simulink model "AUAV_V3_TestSensors"  (R2015a)
settings: Solver=FixedStepDiscrete  StartTime=0.0  StopTime=10.0  FixedStep=T  RelTol=1e-3
PreLoadFcn:
  | %T = 0.0025;
  | MavlinkBus;
  | mcuInit;
  | % Baro Altitude Computation
  | % =========================
  | basePressure = 98192.64;
  | baseTemp = 288.215;
  | lapseRate = -0.00198122;
  | baseHeight = 0;
undefined symbols (not defined in the file): A0, A14, A15, A2, A3, A4, A5, A6, accBiasRateLimit, apSampleTime, B0, bankCommandLimit, barAdjust, baroCutoff, baroCutTemp, baroOffset, baroScale, barTGain1, barTGain2, barTMean1, barTMean2, bda, bde, bdr, bdt, bICda, bICde, bICdr, bICdt, cubeAccelGain16405, cubeGyroGain16405, cubeMagGain16405, D0, D11, D7, D8, daLimit, data, daTrimMax, daTrimMin, deLimit, derivativesConstant, deTrimMax, deTrimMin, drLimit, drTrimMax, drTrimMin, dtLimit, dtTrimMax, dtTrimMin, F2, F3, G0, G13, G15, gaind, GS_location, gyroBiasRateLimit, IC1max, imuOffset_xacc ... (+77)
libraries: MCHP_Blockset x158, simulink x84, SLUGS_Library x31, aerolibconvert2 x6, aerolibutil x4, aerolibtransform2 x3, dspmtrx3 x2, aerolibobsolete x2
(part 13 of 23)

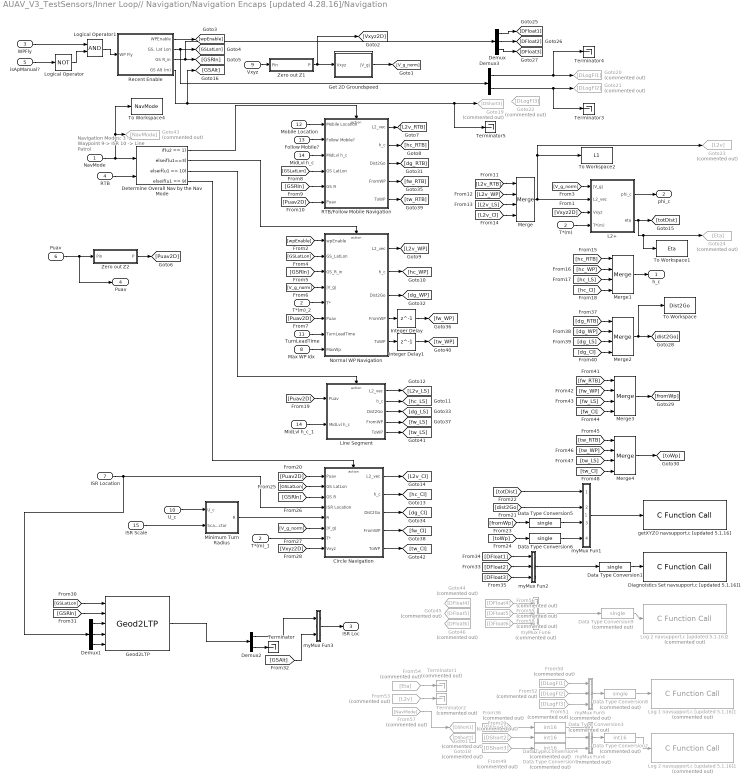
== system AUAV_V3_TestSensors/Inner Loop// Navigation/Navigation Encaps [updated 4.28.16]/Navigation ==
  note: Navigation Modes:
      | 3 -> Waypoint
      | 9-> ISR
      | 10 -> Line Patrol
  NavMode : Inport
  T*(m) : Inport  Port=2
  WPFly : Inport  Port=3
  RTB : Inport  Port=4
  isApManual? : Inport  Port=5
  Puav : Inport  Port=6  SampleTime=apSampleTime
  ISR Location : Inport  Port=7
  Max WP Idx : Inport  Port=8
  Vxyz : Inport  Port=9  SampleTime=apSampleTime
  U_c : Inport  Port=10
  TurnLeadTime : Inport  Port=11
  Mobile Location : Inport  Port=12
  Follow Mobile? : Inport  Port=13
  MidLvl h_c : Inport  Port=14
  ISR Scale : Inport  Port=15
  Circle Navigation : Subsystem  TreatAsAtomicUnit=on
  Data Type Conversion1 : DataTypeConversion  OutDataTypeStr=single
  Data Type Conversion{2..4,7} (4 alike) : DataTypeConversion  Commented=on  OutDataTypeStr=int16
  Data Type Conversion5 : DataTypeConversion  OutDataTypeStr=single
  Data Type Conversion6 : DataTypeConversion  OutDataTypeStr=single
  Data Type Conversion8 : DataTypeConversion  Commented=on  OutDataTypeStr=single
  Data Type Conversion9 : DataTypeConversion  Commented=on  OutDataTypeStr=single
  Demux : Demux  Outputs=3
  Demux1 : Demux  Outputs=3
  Demux2 : Demux  Outputs=[2 1]
  Demux3 : Demux  Outputs=2
  Determine Overall Nav by the Nav Mode : If  NumInputs=2  IfExpression=u2 == 1  ElseIfExpressions=u1==3, u1 == 10, u1 == 9  ShowElse=off
  Diagnoistics Set navsupport.c [updated 5.1.16]1 : MCHP_Blockset/User Functions/C Function Call  ParseFilesChkbx=off  ListFunctions1=Custom Function  Function1=void setDiagnosticFloat(float * flValues)  AddHeaderDeclaration=on  Function1Type=when block is updated (default)  Fct1BlockIn=flValues  FctReturnBlockOut=on  DataCollected=0  ORDERING=None  SampleTime=-1  MCHP_MASTERLINK=|  PinDigitalInput=[]  PinDigitalOutput=[]  PinAnalogInput=[]
      | AUAV_V3_TestSensors/Microchip Master
      | AUAV V3 Board
      | Busy Flag on D2 (RA6)
  From29 : From  Commented=on  GotoTag=DShort2
  From36 : From  Commented=on  GotoTag=DShort1
  From49 : From  Commented=on  GotoTag=DShort3
  From50 : From  Commented=on  GotoTag=DLogFl1
  From51 : From  Commented=on  GotoTag=DLogFl3
  From52 : From  Commented=on  GotoTag=DLogFl2
  From53 : From  Commented=on  GotoTag=L2v
  From54 : From  Commented=on  GotoTag=Eta
  From55 : From  Commented=on  GotoTag=DFloat5
  From56 : From  Commented=on  GotoTag=DFloat4
  From57 : From  Commented=on  GotoTag=NavMode
  From58 : From  Commented=on  GotoTag=DFloat6
  Geod2LTP : SLUGS_Library/Navigation/Geod2LTP
  Get 2D Groundspeed : Subsystem
  Goto17 : Goto  Commented=on  GotoTag=DShort1
  Goto18 : Goto  Commented=on  GotoTag=DShort2
  Goto19 : Goto  Commented=on  GotoTag=DShort3
  Goto20 : Goto  Commented=on  GotoTag=DLogFl1
  Goto21 : Goto  Commented=on  GotoTag=DLogFl2
  Goto22 : Goto  Commented=on  GotoTag=DLogFl3
  Goto23 : Goto  Commented=on  GotoTag=L2v
  Goto24 : Goto  Commented=on  GotoTag=Eta
  Goto43 : Goto  Commented=on  GotoTag=NavMode
  Goto44 : Goto  Commented=on  GotoTag=DFloat4
  Goto45 : Goto  Commented=on  GotoTag=DFloat5
  Goto46 : Goto  Commented=on  GotoTag=DFloat6
  Integer Delay : Delay  DelayLength=1  InputProcessing=Inherited
  Integer Delay1 : Delay  DelayLength=1  InputProcessing=Inherited
  L2+ : Subsystem
  Line Segment : Subsystem  TreatAsAtomicUnit=on
  Log 1 navsupport.c [updated 5.1.16]1 : MCHP_Blockset/User Functions/C Function Call  Commented=on  ParseFilesChkbx=off  ListFunctions1=Custom Function  Function1=void setDiagnosticFloat(float * flValues)  AddHeaderDeclaration=on  Function1Type=when block is updated (default)  Fct1BlockIn=flValues  FctReturnBlockOut=on  DataCollected=0  ORDERING=None  SampleTime=-1  MCHP_MASTERLINK=|  PinDigitalInput=[]  PinDigitalOutput=[]  PinAnalogInput=[]
      | AUAV_V3_TestSensors/Microchip Master
      | AUAV V3 Board
      | Busy Flag on D2 (RA6)
  Log 2 navsupport.c [updated 5.1.16]1 : MCHP_Blockset/User Functions/C Function Call  Commented=on  ParseFilesChkbx=off  ListFunctions1=Custom Function  Function1=void setDiagnosticShort(int16_t *shValues)  AddHeaderDeclaration=on  Function1Type=when block is updated (default)  Fct1BlockIn=shValues  FctReturnBlockOut=on  DataCollected=0  ORDERING=None  SampleTime=-1  MCHP_MASTERLINK=|  PinDigitalInput=[]  PinDigitalOutput=[]  PinAnalogInput=[]
      | AUAV_V3_TestSensors/Microchip Master
      | AUAV V3 Board
      | Busy Flag on D2 (RA6)
  Log 2 navsupport.c [updated 5.1.16]2 : MCHP_Blockset/User Functions/C Function Call  Commented=on  ParseFilesChkbx=off  ListFunctions1=Custom Function  Function1=void setDiagnosticFloat(float * flValues)  AddHeaderDeclaration=on  Function1Type=when block is updated (default)  Fct1BlockIn=flValues  FctReturnBlockOut=on  DataCollected=0  ORDERING=None  SampleTime=-1  MCHP_MASTERLINK=|  PinDigitalInput=[]  PinDigitalOutput=[]  PinAnalogInput=[]
      | AUAV_V3_TestSensors/Microchip Master
      | AUAV V3 Board
      | Busy Flag on D2 (RA6)
  Logical Operator : Logic  Operator=NOT  AllPortsSameDT=off  OutDataTypeStr=boolean
  Logical Operator1 : Logic  AllPortsSameDT=off  OutDataTypeStr=boolean
  Merge{,1..4} (5 alike) : Merge  Inputs=4
  MidLvl h_c_1 : InportShadow  Port=14
  Minimum Turn Radius : Subsystem
  Normal WP Navigation : Subsystem  TreatAsAtomicUnit=on
  RTB/Follow Mobile Navigation : Subsystem
  Recent Enable : Subsystem
  T*(m)_1 : InportShadow  Port=2
  T*(m)_2 : InportShadow  Port=2
  Terminator{,3..5} (4 alike) : Terminator
  Terminator1 : Terminator  Commented=on
  Terminator2 : Terminator  Commented=on
  To Workspace : ToWorkspace  VariableName=Dist2Go  SampleTime=-1
  To Workspace1 : ToWorkspace  VariableName=Eta  SampleTime=-1
  To Workspace2 : ToWorkspace  VariableName=L1  SampleTime=-1
  To Workspace4 : ToWorkspace  VariableName=NavMode  SampleTime=-1
  Zero out Z1 : MATLAB Function  TreatAsAtomicUnit=on
  Zero out Z2 : MATLAB Function  TreatAsAtomicUnit=on
  getXYZ() navsupport.c [updated 5.1.16] : MCHP_Blockset/User Functions/C Function Call  ParseFilesChkbx=on  ListFunctions1=Custom Function  Function1=void setNavNav(float* values)  AddHeaderDeclaration=on  Function1Type=when block is updated (default)  Fct1BlockIn=values  FctReturnBlockOut=on  DataCollected="s.chksm=reshape({ '638529-אוק-2016 01:00:36','251929-אוק-2016 01:00:36','1689429-אוק-2016 01:00:36','4250714-אוק-2016 08:45:05','360329-אוק-2016 01:00:36','7293729-אוק-2016 01:00:36','954929-אוק-2016 01:00:36','296129-אוק-2016 01:00:36','278129-אוק-2016 01:00:36','556029-אוק-2016 01:00:36','963229-אוק-2016 01:00:36','1122729-אוק-2016 01:00:36','372429-אוק-2016 01:00:36','998829-אוק-2016 01:00:36','536514-אוק-2016 08:45:05'},1,15);s.File1=reshape({ '  void  newCircBuffer(CBRef cB)','  void  freeCircBuffer(CBRef* cB)','  void  freeCircBuffer(CBRef* cB)',' unsigned int  getLength(CBRef cB)','  int  readHead(CBRef cB)','  int  readTail(CBRef cB)',' unsigned char  peak(CBRef cB)',' unsigned char  readFront(CBRef cB)',' unsigned char  writeBack(CBRef cB, unsigned char data)','  void  makeEmpty(CBRef cB)','  void  printCircBuf(CBRef cB)'},1,11);s.File2=reshape({ '  void  uartBufferInit(void)','  void  __attribute__((__interrupt__, no_auto_psv)) _U4RXInterrupt(void)','  void  getGPSRawData(unsigned char* gpsBuffer)',' unsigned char  isGPSNovatel(void)'},1,4);s.File3=reshape({ '  char  hex2char(char halfhex)','  float  degMinToDeg(unsigned char degrees, float minutes)',' unsigned char  gpsUbloxSeparate(unsigned char* outStream)','  void  gpsUbloxParse(void)','  void  getGpsUbloxMainData(float* data)','  void  getGpsUbloxData(float* data)','  char  gpSmbl(char symbl)',' unsigned char  myTokenizer(char* stringToTokenize, char token, char * returnToken)','  void  parseRMC(unsigned char* stream)','  void  parseGGA(unsigned char* stream)',' unsigned char  getChecksum(unsigned char* sentence, unsigned char size)','  void  gpsDebugMsg(unsigned char buf)'},1,12);s.File4=reshape({ '  void  uartMavlinkBufferInit(void)','  void __attribute__((__interrupt__,__auto_psv__)) _U1RXInterrupt(void)','  uint8_t  isFinite(float s)','  void  InitParameterInterface(void)','  void  protDecodeMavlink(void)','  uint16_t  MissionInterfaceResponse(uint8_t system_id, uint8_t component_id)','  uint16_t  ParameterInterfaceResponse(uint8_t system_id, uint8_t component_id)','  uint16_t  PackHeartBeat(uint8_t system_id, uint8_t component_id)','  uint16_t  PackTextMsg(uint8_t system_id, uint8_t component_id, unsigned char buf)','  uint16_t  PackRawIMU(uint8_t system_id, uint8_t component_id, mavlink_raw_imu_t mlRawIMUData ,uint32_t time_usec)','  uint16_t  PackRawAttitude(uint8_t system_id, uint8_t component_id, mavlink_attitude_t mlAttitudeData ,uint32_t time_usec)','  uint16_t  PackPosXYZ_Sol(uint8_t system_id, uint8_t component_id, mavlink_local_position_ned_t mlLocalPositionSol ,uint32_t time_usec)','  uint16_t  PackGpsRawInt(uint8_t system_id, uint8_t component_id, mavlink_gps_raw_int_t mlRawGpsDataInt ,uint32_t time_usec)','  uint16_t  PackScaledPressure(uint8_t system_id, uint8_t component_id, mavlink_scaled_pressure_t mlAirData ,uint32_t time_usec)','  uint16_t  PackSysStatus(uint8_t system_id, uint8_t component_id, mavlink_sys_status_t mlSysStatus)','  uint16_t  PackRawServo(uint8_t system_id, uint8_t component_id, mavlink_servo_output_raw_t mlPwmCommands ,uint32_t time_usec)','  uint16_t  HIL_PackRawServo(uint8_t system_id, uint8_t component_id, mavlink_servo_output_raw_t mlPwmCommands ,uint32_t time_usec)','  uint16_t  PackRawRC(uint8_t system_id, uint8_t component_id, mavlink_rc_channels_raw_t mlRC_Commands ,uint32_t time_usec)','  uint16_t  PackVFR_HUD(uint8_t system_id, uint8_t component_id, mavlink_vfr_hud_t mlVfr_hud ,uint32_t time_usec)','  char  sendQGCDebugMessage(const char * dbgMessage, char severity, unsigned char* bytesToAdd, char positionStart)','  void  TxN_Data_OverU1(uint16_t N)','  void  TxN_Data_OverU4(uint16_t N)'},1,22);s.File5=reshape({ '  float  myAtan2(float num, float denom)','  float  myPow(float x, float toTheN)','  float  mySqrt(float x)','  float  myAbs(float x)','  float  myAtan(float x)','  float  myAsin(float x)','  float  mySin(float x)','  float  myCos(float x)','  float  myTan(float x)','  float  myAcos(float x)','  float  myExp(float x)','  void  hugeDelay(void)','  void  smallDelay(void)','  void  tinyDelay(void)','  void  printToUart2(const char *fmt, ...)'},1,15);s.File6=reshape({ '  void  sendTelemetryMavlink(unsigned char* dataOut)','  void  uart2Init(void)','  void  gsRead(unsigned char* gsChunk)','  void  prepareTelemetryMavlink(unsigned char* dataOut)','  void  prepareTelemetryMavlink(unsigned char* dataOut)','  void  sendTelemetryMavlink(unsigned char* dataOut)','  void  copyBufferToDMA1(unsigned char size)','  void  send2GS(unsigned char* protData)','  uint8_t  clearWaypointsFrom(uint8_t startingWp)','  void  addMessageToSpiOut(mavlink_message_t* msg)'},1,10);s.File7={ '  void  populateParameterInterface(void)'};s.File8={ '  void  mavlinkInit(void)'};s.File9=reshape({ '  void  updatePWM(unsigned short * PWMData)','  void  updatePWMTrim(unsigned short PWMData, unsigned char channel)','  void  updateLoad(uint8_t mcuLoad)','  void  updateEuler(float* newEuler)','  void  updatePQR(float* newPQR)',' unsigned char  getHilOnOff(void)','  uint8_t  getLightsOnOff(void)','  uint8_t  getLightsDayNight(void)','  void  updateVISensor(uint16_t* data)','  void  updatePTZ(int16_t* ptz)'},1,10);s.File10=reshape({ '  void  updateRawADCData(int16_t* adcData)','  void  updateAirData(float* airData)','  void  updateLoadData(uint8_t load, uint16_t mvPower)','  void  updateAttitude(float * attitudeData)','  void  getGSLocation(float* altLatLon)','  void  updateTimeStamp(uint32_t timeSt)','  void  updatePosition(float * posData)','  void  updatePilotConsole(uint16_t * pilData)','  void  updateDiagnosticFl(float* diagFl)','  void  updateDiagnosticSh(int16_t* diagSh)','  void  updateBias(float * biasData)','  void  updateSensorData(float* sens)','  uint8_t  isFixValid(void)','  void  updateSensorDiag(float* diag)'},1,14);s.File11=reshape({ '  void  gpsInit(void)','  void  gpsParse(uint8_t* dataStream)','  void  updateStatus(uint8_t* completeMessage)','  void  updatePositionData(uint8_t* completeMessage)','  void  updateVelocityData(uint8_t* completeMessage)','  void  updateTimeData(uint8_t* completeMessage)','  void  getGpsMainData(float* data)','  uint32_t  CRC32Value(int32_t i)','  uint32_t  CalculateBlockCRC32(uint32_t ulCount, uint8_t *ucBuffer)','  uint16_t  charsToUint16(uint8_t* data)','  uint32_t  charsToUint32(uint8_t* data)','  float  charsToFloat(uint8_t* data)','  double  charsToDouble(uint8_t* data)'},1,13);s.File12=reshape({ '  void  getMidLevelCommands(float* commands)',' unsigned char  isApManual(uint16_t failsafe)','  float  getParamIdx(unsigned char idx)','  void  getRangeOfParams(uint8_t startIdx, uint8_t endIdx, float* parameters)','  float  getDynamic(void)','  void  getAttitude(float* attitude)','  void  getXYZ(float* xyz)','  void  getVned(float* xyz)','  uint8_t  getMaxWp(void)',' unsigned char  isWpFly(void)',' unsigned char  isPassthrough(void)','  void  setDiagnosticFloat(float * flValues)','  void  setDiagnosticShort(int16_t* shValues)','  void  getWP(unsigned char idx, float* WPpos)','  void  setLogFloat1(float * flValues)','  void  setLogFloat2(float * flValues)',' unsigned char  getApControlType(void)',' unsigned char  getPassValues(uint8_t* pasVals)','  void  setCurrentCommands(float airSpeed)','  void  getCurrentGPSPos(float* latLonAlt)','  void  setNavLong(float* values)','  void  setNavLat(float* values)','  void  setNavNav(float* values)','  void  getAccels(float * accels)','  void  getAccBias(float * bias)','  void  getRTB(uint8_t* rtb)','  void  getMobileLocation(float* loc)','  uint8_t  getNavMode(void)','  void  getISRLocation(float* loc)','  uint8_t  getISRCameraOption1(void)',' unsigned short  meanFilter5(unsigned short * values)','  uint8_t  justEnabled(uint8_t enableValue, uint8_t index)',' unsigned char  quickSort(unsigned short *arr, char elements)'},1,33);s.File13=reshape({ '  void  hilRead(unsigned char* hilChunk)','  void  hil_getRawRead(short * rawData)','  void  hil_getVned(float* vned)','  void  hil_getEuler(float* euler)','  void  hil_getRates(float* pqr)','  void  hil_getXYZ(float* xyz)',' unsigned int  hil_getTs(void)','  void  protDecodeHil(uint8_t* dataIn)'},1,8);s.File14=reshape({ '  void  cubeInit(void)','  void  getCubeData(short * cubeData)','  void  updateCubeData(void)','  int16_t  averageData(int16_t* theData, uint8_t count)',' unsigned short  write2Cube(unsigned short data2Send)','  short  convert14BitToShort(short wordData)','  short  convert12BitToShort(short wordData)',' unsigned char  isCube16405(void)'},1,8);s.File15=reshape({ '  void  uartMavlinkBufferInit(void)','  uint16_t  PackHeartBeat(uint8_t system_id, uint8_t component_id)','  uint16_t  PackRawServo(uint8_t system_id, uint8_t component_id, mavlink_servo_output_raw_t mlPwmCommands ,uint32_t time_usec)','  uint16_t  HIL_PackRawServo(uint8_t system_id, uint8_t component_id, mavlink_servo_output_raw_t mlPwmCommands ,uint32_t time_usec)','  uint16_t  PackRawRC(uint8_t system_id, uint8_t component_id, mavlink_rc_channels_raw_t mlRC_Commands, uint32_t time_usec)','  uint16_t  PackVFR_HUD(uint8_t system_id, uint8_t component_id, mavlink_vfr_hud_t mlVfr_hud, uint32_t time_usec)','  uint16_t  PackRawIMU(uint8_t system_id, uint8_t component_id, mavlink_raw_imu_t mlRawIMUData ,uint32_t time_usec)','  uint16_t  PackRawAttitude(uint8_t system_id, uint8_t component_id, mavlink_attitude_t mlAttitudeData ,uint32_t time_usec)','  uint16_t  PackPosXYZ_Sol(uint8_t system_id, uint8_t component_id, mavlink_local_position_ned_t mlLocalPositionSol ,uint32_t time_usec)','  char  sendQGCDebugMessage(const char * dbgMessage, char severity, unsigned char* bytesToAdd, char positionStart)','  uint16_t  PackGpsRawInt(uint8_t system_id, uint8_t component_id, mavlink_gps_raw_int_t mlRawGpsDataInt, uint32_t time_usec)','  uint16_t  PackScaledPressure(uint8_t system_id, uint8_t component_id, mavlink_scaled_pressure_t mlAirData, uint32_t time_usec)','  uint16_t  PackSysStatus(uint8_t system_id, uint8_t component_id, mavlink_sys_status_t mlSysStatus)'},1,13);"  ORDERING=None  SampleTime=-1  MCHP_MASTERLINK=|  PinDigitalInput=[]  PinDigitalOutput=[]  PinAnalogInput=[]
      | AUAV_V3_TestSensors/Microchip Master
      | AUAV V3 Board
      | Busy Flag on D2 (RA6)
  myMux Fun1 : MATLAB Function  TreatAsAtomicUnit=on
  myMux Fun2 : MATLAB Function  TreatAsAtomicUnit=on
  myMux Fun3 : MATLAB Function  TreatAsAtomicUnit=on
  myMux Fun4 : MATLAB Function  Commented=on  TreatAsAtomicUnit=on
  myMux Fun5 : MATLAB Function  Commented=on  TreatAsAtomicUnit=on
  myMux Fun6 : MATLAB Function  Commented=on  TreatAsAtomicUnit=on
  h_c : Outport
  phi_c : Outport  Port=2
  ISR Loc : Outport  Port=3
  "Puav " : Outport  Port=4
  wires:
  Data Type Conversion8/1 -> Log 1 navsupport.c [updated 5.1.16]1/1
  From50/1 -> myMux Fun5/1(u1)
  From52/1 -> myMux Fun5/2(u2)
  From51/1 -> myMux Fun5/3(u3)
  myMux Fun5/1(y) -> Data Type Conversion8/1
  Data Type Conversion7/1 -> myMux Fun4/3(u3)
  Data Type Conversion4/1 -> myMux Fun4/2(u2)
  Data Type Conversion3/1 -> myMux Fun4/1(u1)
  From49/1 -> Data Type Conversion7/1
  From36/1 -> Data Type Conversion3/1
  From29/1 -> Data Type Conversion4/1
  myMux Fun4/1(y) -> Data Type Conversion2/1
  Data Type Conversion2/1 -> Log 2 navsupport.c [updated 5.1.16]1/1
  [GSAlt] -> myMux Fun3/2(u2)
  Geod2LTP/1 -> Demux2/1
  Demux2/2 -> Terminator/1
  Demux2/1 -> myMux Fun3/1(u1)
  myMux Fun3/1(y) -> ISR Loc/1
  [GSRIn] -> Geod2LTP/2
  [GSLatLon] -> Geod2LTP/1
  Demux1/3 -> Geod2LTP/5
  Demux1/2 -> Geod2LTP/4
  Demux1/1 -> Geod2LTP/3
  Data Type Conversion1/1 -> Diagnoistics Set navsupport.c [updated 5.1.16]1/1
  [DFloat3] -> myMux Fun2/3(u3)
  [DFloat1] -> myMux Fun2/1(u1)
  [DFloat2] -> myMux Fun2/2(u2)
  ISR Scale/1 -> Minimum Turn Radius/2(Scale Factor)
  U_c/1 -> Minimum Turn Radius/1(U_c)
  ISR Location/1 -> Demux1/1, Circle Navigation/4(ISR Location)
  [Vxyz2D] -> Circle Navigation/8(Vxyz)
  T*(m)_1/1 -> Circle Navigation/7(T*)
  [V_g_norm] -> Circle Navigation/6(|V_g|)
  Minimum Turn Radius/1(R) -> Circle Navigation/5(R)
  [GSRIn] -> Circle Navigation/3(GS R)
  [GSLatLon] -> Circle Navigation/2(GS LatLon)
  Circle Navigation/5(ToWP) -> [tw_CI]
  Circle Navigation/4(FromWP) -> [fw_CI]
  Circle Navigation/3(Dist2Go) -> [dg_CI]
  Circle Navigation/1(L2_vec) -> [L2v_CI]
  Circle Navigation/2(h_c) -> [hc_CI]
  [Puav2D] -> Circle Navigation/1(Puav)
  Integer Delay1/1 -> [tw_WP]
  Integer Delay/1 -> [fw_WP]
  Line Segment/5(ToWP) -> [tw_LS]
  Normal WP Navigation/5(ToWP) -> Integer Delay1/1
  RTB/Follow Mobile Navigation/5(ToWP) -> [tw_RTB]
  Line Segment/4(FromWP) -> [fw_LS]
  Normal WP Navigation/4(FromWP) -> Integer Delay/1
  RTB/Follow Mobile Navigation/4(FromWP) -> [fw_RTB]
  Line Segment/3(Dist2Go) -> [dg_LS]
  Normal WP Navigation/3(Dist2Go) -> [dg_WP]
  RTB/Follow Mobile Navigation/3(Dist2Go) -> [dg_RTB]
  Merge3/1 -> [fromWp]
  Merge4/1 -> [toWp]
  Merge2/1 -> [dist2Go], To Workspace/1
  [tw_RTB] -> Merge4/1
  [tw_WP] -> Merge4/2
  [tw_LS] -> Merge4/3
  [tw_CI] -> Merge4/4
  [fw_RTB] -> Merge3/1
  [fw_WP] -> Merge3/2
  [fw_LS] -> Merge3/3
  [fw_CI] -> Merge3/4
  [dg_RTB] -> Merge2/1
  [dg_WP] -> Merge2/2
  [dg_LS] -> Merge2/3
  [dg_CI] -> Merge2/4
  L2+/2(eta) -> [totDist], Goto24/1, To Workspace1/1
  Data Type Conversion6/1 -> myMux Fun1/4(u4)
  Data Type Conversion5/1 -> myMux Fun1/3(u3)
  [toWp] -> Data Type Conversion6/1
  [fromWp] -> Data Type Conversion5/1
  [dist2Go] -> myMux Fun1/2(u2)
  [totDist] -> myMux Fun1/1(u1)
  myMux Fun1/1(y) -> getXYZ() navsupport.c [updated 5.1.16]/1
  Vxyz/1 -> Zero out Z1/1(Pin)
  Get 2D Groundspeed/1(|V_g|) -> [V_g_norm]
  [Vxyz2D] -> L2+/3(Vxyz)
  [V_g_norm] -> L2+/1(|V_g|)
  L2+/1(phi_c) -> phi_c/1
  T*(m)/1 -> L2+/4(T*(m))
  NavMode/1 -> Determine Overall Nav by the Nav Mode/1, Goto43/1, To Workspace4/1
  Merge/1 -> L2+/2(L2_vec), Goto23/1, To Workspace2/1
  Recent Enable/1(WPEnable) -> [wpEnable]
  Recent Enable/2("GS, Lat Lon") -> [GSLatLon], Demux3/1
  Recent Enable/3(GS R_in) -> [GSRIn], Demux/1
  RTB/1 -> Determine Overall Nav by the Nav Mode/2
  Follow Mobile?/1 -> RTB/Follow Mobile Navigation/2(Follow Mobile?)
  MidLvl h_c/1 -> RTB/Follow Mobile Navigation/3(MidLvl h_c)
  Mobile Location/1 -> RTB/Follow Mobile Navigation/1(Mobile Location)
  Zero out Z1/1(P) -> Get 2D Groundspeed/1(Vxyz), [Vxyz2D]
  Puav/1 -> "Puav "/1, Zero out Z2/1(Pin)
  [GSRIn] -> Normal WP Navigation/3(GS_R_in)
  [GSLatLon] -> Normal WP Navigation/2(GS_LatLon)
  [wpEnable] -> Normal WP Navigation/1(wpEnable)
  [V_g_norm] -> Normal WP Navigation/4(|V_g|)
  T*(m)_2/1 -> Normal WP Navigation/5(T*)
  [Puav2D] -> Normal WP Navigation/6(Puav)
  TurnLeadTime/1 -> Normal WP Navigation/7(TurnLeadTime)
  Max WP Idx/1 -> Normal WP Navigation/8(MaxWp)
  [GSLatLon] -> RTB/Follow Mobile Navigation/4(GS LatLon)
  [GSRIn] -> RTB/Follow Mobile Navigation/5(GS R)
  Zero out Z2/1(P) -> [Puav2D]
  [Puav2D] -> RTB/Follow Mobile Navigation/6(Puav)
  Merge1/1 -> h_c/1
  RTB/Follow Mobile Navigation/1(L2_vec) -> [L2v_RTB]
  RTB/Follow Mobile Navigation/2(h_c) -> [hc_RTB]
  Normal WP Navigation/1(L2_vec) -> [L2v_WP]
  Normal WP Navigation/2(h_c) -> [hc_WP]
  Line Segment/1(L2_vec) -> [L2v_LS]
  Line Segment/2(h_c) -> [hc_LS]
  [L2v_RTB] -> Merge/1
  [L2v_WP] -> Merge/2
  [L2v_LS] -> Merge/3
  [L2v_CI] -> Merge/4
  [hc_RTB] -> Merge1/1
  [hc_WP] -> Merge1/2
  [hc_LS] -> Merge1/3
  [hc_CI] -> Merge1/4
  [Puav2D] -> Line Segment/1(Puav)
  MidLvl h_c_1/1 -> Line Segment/2(MidLvl h_c)
  isApManual?/1 -> Logical Operator/1
  Logical Operator1/1 -> Recent Enable/1(WP Fly)
  Logical Operator/1 -> Logical Operator1/2
  WPFly/1 -> Logical Operator1/1
  myMux Fun2/1(y) -> Data Type Conversion1/1
  From54/1 -> Terminator1/1
  From53/1 -> Terminator2/1
  Demux/1 -> [DFloat1]
  Demux/2 -> [DFloat2]
  Demux3/1 -> Terminator4/1, Goto20/1
  Demux3/2 -> Terminator3/1, Goto21/1
  From57/1 -> Goto17/1
  Demux/3 -> [DFloat3]
  Recent Enable/4(GS Alt (m)) -> Terminator5/1, Goto19/1, [GSAlt]
  From58/1 -> myMux Fun6/3(u3)
  From56/1 -> myMux Fun6/1(u1)
  From55/1 -> myMux Fun6/2(u2)
  myMux Fun6/1(y) -> Data Type Conversion9/1
  Data Type Conversion9/1 -> Log 2 navsupport.c [updated 5.1.16]2/1
  Determine Overall Nav by the Nav Mode/1 -> RTB/Follow Mobile Navigation/Action
  Determine Overall Nav by the Nav Mode/2 -> Normal WP Navigation/Action
  Determine Overall Nav by the Nav Mode/3 -> Line Segment/Action
  Determine Overall Nav by the Nav Mode/4 -> Circle Navigation/Action

== system AUAV_V3_TestSensors/Position_and_Attitude_Filter/Attitude Complimentary Filter COG/3D Filter ==
  In1 : Inport
  Data Type Conversion1 : DataTypeConversion  OutDataTypeStr=single
  Data Type Conversion2 : DataTypeConversion  OutDataTypeStr=double
  Demux : Demux  Outputs=3
  Filter1 : Subsystem  mask(DiscretizedZeroPole){Zeros=zval, Poles=pval, Gain=kval, AbsTol=auto, SampleTime=TSample, method=tustin, Wc=1}
      mask prompts: Zeros "Zeros (enter in s-main:)"; Poles "Poles (enter in s-domain:)"; Gain "Gain (enter in s-domain:)"; AbsTol "Absolute tolerance:"; SampleTime "Sample time:"; Wc "Critical Frequency (Hz):"
      mask help: Continuous mask uses c2d to transform parameters onto the Discrete Zero-Pole block inside.
      mask init: same as AUAV_V3_TestSensors/Barometer_Driver/Baro Altimeter/Initial Baro Bias/Low Pass8
      mask TypeOptions method: zoh | foh | tustin | prewarp | matched
      mask Callback method: hidecrit
      mask Display:
      | droots(zeross,poless,gainss)
      | text( 0.5, 1.0, method, 'verticalAlignment','top')
  Filter2 : Subsystem  mask(DiscretizedZeroPole){Zeros=zval, Poles=pval, Gain=kval, AbsTol=auto, SampleTime=TSample, method=tustin, Wc=1}
      mask prompts: Zeros "Zeros (enter in s-main:)"; Poles "Poles (enter in s-domain:)"; Gain "Gain (enter in s-domain:)"; AbsTol "Absolute tolerance:"; SampleTime "Sample time:"; Wc "Critical Frequency (Hz):"
      mask help: Continuous mask uses c2d to transform parameters onto the Discrete Zero-Pole block inside.
      mask init: same as AUAV_V3_TestSensors/Barometer_Driver/Baro Altimeter/Initial Baro Bias/Low Pass8
      mask TypeOptions method: zoh | foh | tustin | prewarp | matched
      mask Callback method: hidecrit
      mask Display:
      | droots(zeross,poless,gainss)
      | text( 0.5, 1.0, method, 'verticalAlignment','top')
  Filter3 : Subsystem  mask(DiscretizedZeroPole){Zeros=zval, Poles=pval, Gain=kval, AbsTol=auto, SampleTime=TSample, method=tustin, Wc=1}
      mask prompts: Zeros "Zeros (enter in s-main:)"; Poles "Poles (enter in s-domain:)"; Gain "Gain (enter in s-domain:)"; AbsTol "Absolute tolerance:"; SampleTime "Sample time:"; Wc "Critical Frequency (Hz):"
      mask help: Continuous mask uses c2d to transform parameters onto the Discrete Zero-Pole block inside.
      mask init: same as AUAV_V3_TestSensors/Barometer_Driver/Baro Altimeter/Initial Baro Bias/Low Pass8
      mask TypeOptions method: zoh | foh | tustin | prewarp | matched
      mask Callback method: hidecrit
      mask Display:
      | droots(zeross,poless,gainss)
      | text( 0.5, 1.0, method, 'verticalAlignment','top')
  myMux Fun1 : MATLAB Function  TreatAsAtomicUnit=on
  Out1 : Outport
  wires:
  myMux Fun1/1(y) -> Data Type Conversion1/1
  In1/1 -> Data Type Conversion2/1
  Filter3/1(Out1) -> myMux Fun1/3(u3)
  Filter2/1(Out1) -> myMux Fun1/2(u2)
  Filter1/1(Out1) -> myMux Fun1/1(u1)
  Demux/3 -> Filter3/1(In1)
  Demux/2 -> Filter2/1(In1)
  Demux/1 -> Filter1/1(In1)
  Data Type Conversion2/1 -> Demux/1
  Data Type Conversion1/1 -> Out1/1

== system AUAV_V3_TestSensors/Position_and_Attitude_Filter/Attitude Complimentary Filter COG/Deriv  ==
  y : Inport
  Gain2 : Gain  Gain=[ 1/(5*apSampleTime) ]
  Integer Delay1 : Delay  DelayLength=5  InitialCondition=double(U_comm)  InputProcessing=Inherited  SampleTime=apSampleTime
  Sum5 : Sum  Inputs=-+|
  ydot : Outport
  wires:
  Sum5/1 -> Gain2/1
  Integer Delay1/1 -> Sum5/1
  y/1 -> Sum5/2, Integer Delay1/1
  Gain2/1 -> ydot/1

== system AUAV_V3_TestSensors/Position_and_Attitude_Filter/Attitude Complimentary Filter COG/Normalize Vector1 ==
  Vector : Inport
  Divide : Product  Inputs=*/
  Norm : Subsystem  AncestorBlock=SLUGS_Library/Navigation/Norm
  Zero Bound : Saturate  UpperLimit=inf  LowerLimit=0.001
  Normalized : Outport
  wires:
  Divide/1 -> Normalized/1
  Zero Bound/1 -> Divide/2
  Norm/1(Norm) -> Zero Bound/1
  Vector/1 -> Divide/1, Norm/1(Vector)

== system AUAV_V3_TestSensors/Position_and_Attitude_Filter/Attitude Complimentary Filter COG/Normalize Vector2 ==
  Vector : Inport
  Divide : Product  Inputs=*/
  Norm : Subsystem  AncestorBlock=SLUGS_Library/Navigation/Norm
  Zero Bound : Saturate  UpperLimit=inf  LowerLimit=0.001
  Normalized : Outport
  wires:
  Vector/1 -> Norm/1(Vector), Divide/1
  Norm/1(Norm) -> Zero Bound/1
  Zero Bound/1 -> Divide/2
  Divide/1 -> Normalized/1

== system AUAV_V3_TestSensors/Position_and_Attitude_Filter/COG.SOG2V/Subsystem5 ==
  u : Inport
  "[apUtils.c]" : MCHP_Blockset/User Functions/C Function Call  ParseFilesChkbx=on  ListFunctions1=Custom Function  Function1=real32_T mySin(real32_T u1);  AddHeaderDeclaration=on  Function1Type=when block is updated (default)  FctReturnBlockOut=on  DataCollected="s.chksm=reshape({ '360325-Apr-2016 19:19:45','638502-Mar-2016 19:06:13','219625-Apr-2016 19:38:33','1593925-Apr-2016 19:41:14','3277826-Apr-2016 00:33:15','294426-Apr-2016 00:47:59','556001-Oct-2014 14:05:42','963201-Apr-2016 12:47:40','358819-Apr-2016 01:35:18','985925-Apr-2016 19:19:45'},1,10);s.File1=reshape({ '  float  myAtan2(float num, float denom)','  float  myPow(float x, float toTheN)','  float  mySqrt(float x)','  float  myAbs(float x)','  float  myAtan(float x)','  float  myAsin(float x)','  float  mySin(float x)','  float  myCos(float x)','  float  myTan(float x)','  float  myAcos(float x)','  float  myExp(float x)','  void  hugeDelay(void)','  void  smallDelay(void)','  void  tinyDelay(void)','  void  printToUart2(const char *fmt, ...)'},1,15);s.File2=reshape({ '  void  newCircBuffer(CBRef cB)','  void  freeCircBuffer(CBRef* cB)','  void  freeCircBuffer(CBRef* cB)',' unsigned int  getLength(CBRef cB)','  int  readHead(CBRef cB)','  int  readTail(CBRef cB)',' unsigned char  peak(CBRef cB)',' unsigned char  readFront(CBRef cB)',' unsigned char  writeBack(CBRef cB, unsigned char data)','  void  makeEmpty(CBRef cB)','  void  printCircBuf(CBRef cB)'},1,11);s.File3=reshape({ '  void  uartBufferInit(void)','  void  __attribute__((__interrupt__, no_auto_psv)) _U4RXInterrupt(void)','  void  getGPSRawData(unsigned char* gpsBuffer)',' unsigned char  isGPSNovatel(void)'},1,4);s.File4=reshape({ '  char  hex2char(char halfhex)','  float  degMinToDeg(unsigned char degrees, float minutes)',' unsigned char  gpsUbloxSeparate(unsigned char* outStream)','  void  gpsUbloxParse(void)','  void  getGpsUbloxMainData(float* data)','  char  gpSmbl(char symbl)',' unsigned char  myTokenizer(char* stringToTokenize, char token, char * returnToken)','  void  parseRMC(unsigned char* stream)','  void  parseGGA(unsigned char* stream)',' unsigned char  getChecksum(unsigned char* sentence, unsigned char size)'},1,10);s.File5=reshape({ '  void  uartMavlinkBufferInit(void)','  void __attribute__((__interrupt__,__auto_psv__)) _U1RXInterrupt(void)','  uint8_t  isFinite(float s)','  void  InitParameterInterface(void)','  void  protDecodeMavlink(void)','  uint16_t  MissionInterfaceResponse(uint8_t system_id, uint8_t component_id)','  uint16_t  ParameterInterfaceResponse(uint8_t system_id, uint8_t component_id)','  uint16_t  PackHeartBeat(uint8_t system_id, uint8_t component_id)','  uint16_t  PackTextMsg(uint8_t system_id, uint8_t component_id)','  uint16_t  PackRawIMU(uint8_t system_id, uint8_t component_id, mavlink_raw_imu_t mlRawIMUData ,uint32_t time_usec)','  uint16_t  PackGpsRawInt(uint8_t system_id, uint8_t component_id, mavlink_gps_raw_int_t mlRawGpsDataInt ,uint32_t time_usec)','  uint16_t  PackScaledPressure(uint8_t system_id, uint8_t component_id, mavlink_scaled_pressure_t mlAirData ,uint32_t time_usec)','  uint16_t  PackSysStatus(uint8_t system_id, uint8_t component_id, mavlink_sys_status_t mlSysStatus)','  char  sendQGCDebugMessage(const char * dbgMessage, char severity, unsigned char* bytesToAdd, char positionStart)','  void  TxN_Data_OverU1(uint16_t N)'},1,15);s.File6={ '  void  mavlinkInit(void)'};s.File7=reshape({ '  void  updateRawADCData(int16_t* adcData)','  void  updateAirData(float* airData)','  void  updateLoadData(uint8_t load, uint16_t mvPower)','  void  updateAttitude(float * attitudeData)','  void  getGSLocation(float* altLatLon)','  void  updateTimeStamp(uint32_t timeSt)','  void  updatePosition(float * posData)','  void  updatePilotConsole(uint16_t * pilData)','  void  updateDiagnosticFl(float* diagFl)','  void  updateDiagnosticSh(int16_t* diagSh)','  void  updateBias(float * biasData)','  void  updateSensorData(float* sens)','  uint8_t  isFixValid(void)','  void  updateSensorDiag(float* diag)'},1,14);s.File8=reshape({ '  void  gpsInit(void)','  void  gpsParse(uint8_t* dataStream)','  void  updateStatus(uint8_t* completeMessage)','  void  updatePositionData(uint8_t* completeMessage)','  void  updateVelocityData(uint8_t* completeMessage)','  void  updateTimeData(uint8_t* completeMessage)','  void  getGpsMainData(float* data)','  uint32_t  CRC32Value(int32_t i)','  uint32_t  CalculateBlockCRC32(uint32_t ulCount, uint8_t *ucBuffer)','  uint16_t  charsToUint16(uint8_t* data)','  uint32_t  charsToUint32(uint8_t* data)','  float  charsToFloat(uint8_t* data)','  double  charsToDouble(uint8_t* data)'},1,13);s.File9=reshape({ '  void  hilRead(unsigned char* hilChunk)','  void  hil_getRawRead(short * rawData)','  void  hil_getVned(float* vned)','  void  hil_getEuler(float* euler)','  void  hil_getRates(float* pqr)','  void  hil_getXYZ(float* xyz)',' unsigned int  hil_getTs(void)','  void  protDecodeHil(uint8_t* dataIn)'},1,8);s.File10=reshape({ '  void  cubeInit(void)','  void  getCubeData(short * cubeData)','  void  updateCubeData(void)','  int16_t  averageData(int16_t* theData, uint8_t count)',' unsigned short  write2Cube(unsigned short data2Send)','  void  __attribute__((interrupt, no_auto_psv)) _T5Interrupt(void)','  short  convert14BitToShort(short wordData)','  short  convert12BitToShort(short wordData)',' unsigned char  isCube16405(void)'},1,9);"  ORDERING=None  SampleTime=-1  MCHP_MASTERLINK=|  PinDigitalInput=[]  PinDigitalOutput=[]  PinAnalogInput=[]
      | AUAV_V3_TestSensors/Microchip Master
      | AUAV V3 Board
      | Busy Flag on D2 (RA6)
  "[apUtils.c]1" : MCHP_Blockset/User Functions/C Function Call  ParseFilesChkbx=on  ListFunctions1=Custom Function  Function1=real32_T myCos(real32_T u1);  AddHeaderDeclaration=on  Function1Type=when block is updated (default)  FctReturnBlockOut=on  DataCollected="s.chksm=reshape({ '638529-אוק-2016 01:00:36','251929-אוק-2016 01:00:36','1689429-אוק-2016 01:00:36','4250714-אוק-2016 08:45:05','360329-אוק-2016 01:00:36','7293729-אוק-2016 01:00:36','954929-אוק-2016 01:00:36','296129-אוק-2016 01:00:36','278129-אוק-2016 01:00:36','556029-אוק-2016 01:00:36','963229-אוק-2016 01:00:36','1122729-אוק-2016 01:00:36','372429-אוק-2016 01:00:36','998829-אוק-2016 01:00:36','536514-אוק-2016 08:45:05'},1,15);s.File1=reshape({ '  void  newCircBuffer(CBRef cB)','  void  freeCircBuffer(CBRef* cB)','  void  freeCircBuffer(CBRef* cB)',' unsigned int  getLength(CBRef cB)','  int  readHead(CBRef cB)','  int  readTail(CBRef cB)',' unsigned char  peak(CBRef cB)',' unsigned char  readFront(CBRef cB)',' unsigned char  writeBack(CBRef cB, unsigned char data)','  void  makeEmpty(CBRef cB)','  void  printCircBuf(CBRef cB)'},1,11);s.File2=reshape({ '  void  uartBufferInit(void)','  void  __attribute__((__interrupt__, no_auto_psv)) _U4RXInterrupt(void)','  void  getGPSRawData(unsigned char* gpsBuffer)',' unsigned char  isGPSNovatel(void)'},1,4);s.File3=reshape({ '  char  hex2char(char halfhex)','  float  degMinToDeg(unsigned char degrees, float minutes)',' unsigned char  gpsUbloxSeparate(unsigned char* outStream)','  void  gpsUbloxParse(void)','  void  getGpsUbloxMainData(float* data)','  void  getGpsUbloxData(float* data)','  char  gpSmbl(char symbl)',' unsigned char  myTokenizer(char* stringToTokenize, char token, char * returnToken)','  void  parseRMC(unsigned char* stream)','  void  parseGGA(unsigned char* stream)',' unsigned char  getChecksum(unsigned char* sentence, unsigned char size)','  void  gpsDebugMsg(unsigned char buf)'},1,12);s.File4=reshape({ '  void  uartMavlinkBufferInit(void)','  void __attribute__((__interrupt__,__auto_psv__)) _U1RXInterrupt(void)','  uint8_t  isFinite(float s)','  void  InitParameterInterface(void)','  void  protDecodeMavlink(void)','  uint16_t  MissionInterfaceResponse(uint8_t system_id, uint8_t component_id)','  uint16_t  ParameterInterfaceResponse(uint8_t system_id, uint8_t component_id)','  uint16_t  PackHeartBeat(uint8_t system_id, uint8_t component_id)','  uint16_t  PackTextMsg(uint8_t system_id, uint8_t component_id, unsigned char buf)','  uint16_t  PackRawIMU(uint8_t system_id, uint8_t component_id, mavlink_raw_imu_t mlRawIMUData ,uint32_t time_usec)','  uint16_t  PackRawAttitude(uint8_t system_id, uint8_t component_id, mavlink_attitude_t mlAttitudeData ,uint32_t time_usec)','  uint16_t  PackPosXYZ_Sol(uint8_t system_id, uint8_t component_id, mavlink_local_position_ned_t mlLocalPositionSol ,uint32_t time_usec)','  uint16_t  PackGpsRawInt(uint8_t system_id, uint8_t component_id, mavlink_gps_raw_int_t mlRawGpsDataInt ,uint32_t time_usec)','  uint16_t  PackScaledPressure(uint8_t system_id, uint8_t component_id, mavlink_scaled_pressure_t mlAirData ,uint32_t time_usec)','  uint16_t  PackSysStatus(uint8_t system_id, uint8_t component_id, mavlink_sys_status_t mlSysStatus)','  uint16_t  PackRawServo(uint8_t system_id, uint8_t component_id, mavlink_servo_output_raw_t mlPwmCommands ,uint32_t time_usec)','  uint16_t  HIL_PackRawServo(uint8_t system_id, uint8_t component_id, mavlink_servo_output_raw_t mlPwmCommands ,uint32_t time_usec)','  uint16_t  PackRawRC(uint8_t system_id, uint8_t component_id, mavlink_rc_channels_raw_t mlRC_Commands ,uint32_t time_usec)','  uint16_t  PackVFR_HUD(uint8_t system_id, uint8_t component_id, mavlink_vfr_hud_t mlVfr_hud ,uint32_t time_usec)','  char  sendQGCDebugMessage(const char * dbgMessage, char severity, unsigned char* bytesToAdd, char positionStart)','  void  TxN_Data_OverU1(uint16_t N)','  void  TxN_Data_OverU4(uint16_t N)'},1,22);s.File5=reshape({ '  float  myAtan2(float num, float denom)','  float  myPow(float x, float toTheN)','  float  mySqrt(float x)','  float  myAbs(float x)','  float  myAtan(float x)','  float  myAsin(float x)','  float  mySin(float x)','  float  myCos(float x)','  float  myTan(float x)','  float  myAcos(float x)','  float  myExp(float x)','  void  hugeDelay(void)','  void  smallDelay(void)','  void  tinyDelay(void)','  void  printToUart2(const char *fmt, ...)'},1,15);s.File6=reshape({ '  void  sendTelemetryMavlink(unsigned char* dataOut)','  void  uart2Init(void)','  void  gsRead(unsigned char* gsChunk)','  void  prepareTelemetryMavlink(unsigned char* dataOut)','  void  prepareTelemetryMavlink(unsigned char* dataOut)','  void  sendTelemetryMavlink(unsigned char* dataOut)','  void  copyBufferToDMA1(unsigned char size)','  void  send2GS(unsigned char* protData)','  uint8_t  clearWaypointsFrom(uint8_t startingWp)','  void  addMessageToSpiOut(mavlink_message_t* msg)'},1,10);s.File7={ '  void  populateParameterInterface(void)'};s.File8={ '  void  mavlinkInit(void)'};s.File9=reshape({ '  void  updatePWM(unsigned short * PWMData)','  void  updatePWMTrim(unsigned short PWMData, unsigned char channel)','  void  updateLoad(uint8_t mcuLoad)','  void  updateEuler(float* newEuler)','  void  updatePQR(float* newPQR)',' unsigned char  getHilOnOff(void)','  uint8_t  getLightsOnOff(void)','  uint8_t  getLightsDayNight(void)','  void  updateVISensor(uint16_t* data)','  void  updatePTZ(int16_t* ptz)'},1,10);s.File10=reshape({ '  void  updateRawADCData(int16_t* adcData)','  void  updateAirData(float* airData)','  void  updateLoadData(uint8_t load, uint16_t mvPower)','  void  updateAttitude(float * attitudeData)','  void  getGSLocation(float* altLatLon)','  void  updateTimeStamp(uint32_t timeSt)','  void  updatePosition(float * posData)','  void  updatePilotConsole(uint16_t * pilData)','  void  updateDiagnosticFl(float* diagFl)','  void  updateDiagnosticSh(int16_t* diagSh)','  void  updateBias(float * biasData)','  void  updateSensorData(float* sens)','  uint8_t  isFixValid(void)','  void  updateSensorDiag(float* diag)'},1,14);s.File11=reshape({ '  void  gpsInit(void)','  void  gpsParse(uint8_t* dataStream)','  void  updateStatus(uint8_t* completeMessage)','  void  updatePositionData(uint8_t* completeMessage)','  void  updateVelocityData(uint8_t* completeMessage)','  void  updateTimeData(uint8_t* completeMessage)','  void  getGpsMainData(float* data)','  uint32_t  CRC32Value(int32_t i)','  uint32_t  CalculateBlockCRC32(uint32_t ulCount, uint8_t *ucBuffer)','  uint16_t  charsToUint16(uint8_t* data)','  uint32_t  charsToUint32(uint8_t* data)','  float  charsToFloat(uint8_t* data)','  double  charsToDouble(uint8_t* data)'},1,13);s.File12=reshape({ '  void  getMidLevelCommands(float* commands)',' unsigned char  isApManual(uint16_t failsafe)','  float  getParamIdx(unsigned char idx)','  void  getRangeOfParams(uint8_t startIdx, uint8_t endIdx, float* parameters)','  float  getDynamic(void)','  void  getAttitude(float* attitude)','  void  getXYZ(float* xyz)','  void  getVned(float* xyz)','  uint8_t  getMaxWp(void)',' unsigned char  isWpFly(void)',' unsigned char  isPassthrough(void)','  void  setDiagnosticFloat(float * flValues)','  void  setDiagnosticShort(int16_t* shValues)','  void  getWP(unsigned char idx, float* WPpos)','  void  setLogFloat1(float * flValues)','  void  setLogFloat2(float * flValues)',' unsigned char  getApControlType(void)',' unsigned char  getPassValues(uint8_t* pasVals)','  void  setCurrentCommands(float airSpeed)','  void  getCurrentGPSPos(float* latLonAlt)','  void  setNavLong(float* values)','  void  setNavLat(float* values)','  void  setNavNav(float* values)','  void  getAccels(float * accels)','  void  getAccBias(float * bias)','  void  getRTB(uint8_t* rtb)','  void  getMobileLocation(float* loc)','  uint8_t  getNavMode(void)','  void  getISRLocation(float* loc)','  uint8_t  getISRCameraOption1(void)',' unsigned short  meanFilter5(unsigned short * values)','  uint8_t  justEnabled(uint8_t enableValue, uint8_t index)',' unsigned char  quickSort(unsigned short *arr, char elements)'},1,33);s.File13=reshape({ '  void  hilRead(unsigned char* hilChunk)','  void  hil_getRawRead(short * rawData)','  void  hil_getVned(float* vned)','  void  hil_getEuler(float* euler)','  void  hil_getRates(float* pqr)','  void  hil_getXYZ(float* xyz)',' unsigned int  hil_getTs(void)','  void  protDecodeHil(uint8_t* dataIn)'},1,8);s.File14=reshape({ '  void  cubeInit(void)','  void  getCubeData(short * cubeData)','  void  updateCubeData(void)','  int16_t  averageData(int16_t* theData, uint8_t count)',' unsigned short  write2Cube(unsigned short data2Send)','  short  convert14BitToShort(short wordData)','  short  convert12BitToShort(short wordData)',' unsigned char  isCube16405(void)'},1,8);s.File15=reshape({ '  void  uartMavlinkBufferInit(void)','  uint16_t  PackHeartBeat(uint8_t system_id, uint8_t component_id)','  uint16_t  PackRawServo(uint8_t system_id, uint8_t component_id, mavlink_servo_output_raw_t mlPwmCommands ,uint32_t time_usec)','  uint16_t  HIL_PackRawServo(uint8_t system_id, uint8_t component_id, mavlink_servo_output_raw_t mlPwmCommands ,uint32_t time_usec)','  uint16_t  PackRawRC(uint8_t system_id, uint8_t component_id, mavlink_rc_channels_raw_t mlRC_Commands, uint32_t time_usec)','  uint16_t  PackVFR_HUD(uint8_t system_id, uint8_t component_id, mavlink_vfr_hud_t mlVfr_hud, uint32_t time_usec)','  uint16_t  PackRawIMU(uint8_t system_id, uint8_t component_id, mavlink_raw_imu_t mlRawIMUData ,uint32_t time_usec)','  uint16_t  PackRawAttitude(uint8_t system_id, uint8_t component_id, mavlink_attitude_t mlAttitudeData ,uint32_t time_usec)','  uint16_t  PackPosXYZ_Sol(uint8_t system_id, uint8_t component_id, mavlink_local_position_ned_t mlLocalPositionSol ,uint32_t time_usec)','  char  sendQGCDebugMessage(const char * dbgMessage, char severity, unsigned char* bytesToAdd, char positionStart)','  uint16_t  PackGpsRawInt(uint8_t system_id, uint8_t component_id, mavlink_gps_raw_int_t mlRawGpsDataInt, uint32_t time_usec)','  uint16_t  PackScaledPressure(uint8_t system_id, uint8_t component_id, mavlink_scaled_pressure_t mlAirData, uint32_t time_usec)','  uint16_t  PackSysStatus(uint8_t system_id, uint8_t component_id, mavlink_sys_status_t mlSysStatus)'},1,13);"  ORDERING=None  SampleTime=-1  MCHP_MASTERLINK=|  PinDigitalInput=[]  PinDigitalOutput=[]  PinAnalogInput=[]
      | AUAV_V3_TestSensors/Microchip Master
      | AUAV V3 Board
      | Busy Flag on D2 (RA6)
  sin(u) : Outport
  cos(u) : Outport  Port=2
  wires:
  u/1 -> "[apUtils.c]"/1, "[apUtils.c]1"/1
  "[apUtils.c]"/1 -> sin(u)/1
  "[apUtils.c]1"/1 -> cos(u)/1

== system AUAV_V3_TestSensors/Position_and_Attitude_Filter/Compute GS Location/Geod2ECEF1 ==
  "height, m" : Inport
  "lat, deg" : Inport  Port=2
  lon,deg : Inport  Port=3
  (Rh+h)cos(phi)*cos(lamb)=Xe : Product  Inputs=3  OutDataTypeStr=single  SaturateOnIntegerOverflow=on  InputSameDT=on
  (Rh+h)cos(phi)*sin(lamb)=Ye : Product  Inputs=3  OutDataTypeStr=single  SaturateOnIntegerOverflow=on  InputSameDT=on
  Deg2R : Gain  Gain=pi/180  OutDataTypeStr=float('single')  SaturateOnIntegerOverflow=on  ParamDataTypeStr=Inherit: Same as input
  Deg2R1 : Gain  Gain=pi/180  OutDataTypeStr=float('single')  SaturateOnIntegerOverflow=on  ParamDataTypeStr=Inherit: Same as input
  Product1 : Product  SaturateOnIntegerOverflow=on  InputSameDT=on  OutDataTypeStr=Inherit: Same as first input
  Re=equatorial radius : Constant  Value=Re  OutDataTypeStr=single
  Rh : Product  Inputs=*/  OutDataTypeStr=single  SaturateOnIntegerOverflow=on  InputSameDT=on
  Rh(1-e^2) : Product  OutDataTypeStr=single  SaturateOnIntegerOverflow=on  InputSameDT=on
  Sum1 : Sum  Inputs=+-|  SaturateOnIntegerOverflow=on  InputSameDT=on  OutDataTypeStr=Inherit: Same as first input
  Sum2 : Sum  SaturateOnIntegerOverflow=on  InputSameDT=on  OutDataTypeStr=Inherit: Same as first input
      settings: AttributesFormatString=Rh+h
  Sum3 : Sum  Inputs=|+-  SaturateOnIntegerOverflow=on  InputSameDT=on  OutDataTypeStr=Inherit: Same as first input
  Sum4 : Sum  OutDataTypeStr=single  SaturateOnIntegerOverflow=on  InputSameDT=on
      settings: AttributesFormatString=(1-e^2)Rh+h
  Ze : Product  OutDataTypeStr=single  SaturateOnIntegerOverflow=on  InputSameDT=on
  const : Constant  OutDataTypeStr=single
  const1 : Constant  OutDataTypeStr=single
  cos(lamb) : Trigonometry  Operator=cos
  cos(phi) : Trigonometry  Operator=cos
  eccentricity^2 : Subsystem
  f : Fcn  Expr=sqrt(u(1))
  sin(lamb) : Trigonometry
  sin(phi) : Trigonometry
  sin(phi)^2 : Product  SaturateOnIntegerOverflow=on  InputSameDT=on  OutDataTypeStr=Inherit: Same as first input
  "Xe, m " : Outport
  "Ye, m " : Outport  Port=2
  "Ze, m " : Outport  Port=3
  wires:
  (Rh+h)cos(phi)*sin(lamb)=Ye/1 -> "Ye, m "/1
  (Rh+h)cos(phi)*cos(lamb)=Xe/1 -> "Xe, m "/1
  Sum2/1 -> (Rh+h)cos(phi)*cos(lamb)=Xe/1, (Rh+h)cos(phi)*sin(lamb)=Ye/1
  Deg2R1/1 -> sin(lamb)/1, cos(lamb)/1
  Deg2R/1 -> sin(phi)/1, cos(phi)/1
  Ze/1 -> "Ze, m "/1
  sin(lamb)/1 -> (Rh+h)cos(phi)*sin(lamb)=Ye/3
  cos(lamb)/1 -> (Rh+h)cos(phi)*cos(lamb)=Xe/3
  cos(phi)/1 -> (Rh+h)cos(phi)*sin(lamb)=Ye/2, (Rh+h)cos(phi)*cos(lamb)=Xe/2
  lon,deg/1 -> Deg2R1/1
  Sum4/1 -> Ze/2
  Rh(1-e^2)/1 -> Sum4/1
  Sum3/1 -> Rh(1-e^2)/1  "1-e^2"
  const1/1 -> Sum3/1
  sin(phi)^2/1 -> Product1/2
  eccentricity^2/1(e^2) -> Sum3/2, Product1/1
  "height, m"/1 -> Sum2/1, Sum4/2
  const/1 -> Sum1/1
  Sum1/1 -> f/1
  Product1/1 -> Sum1/2
  Rh/1 -> Rh(1-e^2)/2, Sum2/2
  Re=equatorial radius/1 -> Rh/1
  f/1 -> Rh/2
  sin(phi)/1 -> Ze/1, sin(phi)^2/2, sin(phi)^2/1
  "lat, deg"/1 -> Deg2R/1

== system AUAV_V3_TestSensors/Position_and_Attitude_Filter/GPS Update/Detect Change ==
  Data : Inport
  Abs1 : Abs  SampleTime=T
  Difference1 : simulink/Discrete/Difference  ICPrevInput=0.0  InputProcessing=Inherited  OutMin=[]  OutMax=[]  OutDataType=sfix(16)  OutScaling=2^-10  DoSatur=off
  Saturation1 : Saturate  UpperLimit=1  LowerLimit=0  SampleTime=T
  change? : Outport
  wires:
  Difference1/1 -> Abs1/1
  Abs1/1 -> Saturation1/1
  Data/1 -> Difference1/1
  Saturation1/1 -> change?/1

== system AUAV_V3_TestSensors/Position_and_Attitude_Filter/GPS Update/Detect Change1 ==
  Data : Inport
  Abs1 : Abs  SampleTime=T
  Difference1 : simulink/Discrete/Difference  ICPrevInput=0.0  InputProcessing=Inherited  OutMin=[]  OutMax=[]  OutDataType=sfix(16)  OutScaling=2^-10  DoSatur=off
  Saturation1 : Saturate  UpperLimit=1  LowerLimit=0  SampleTime=T
  change? : Outport
  wires:
  Saturation1/1 -> change?/1
  Data/1 -> Difference1/1
  Abs1/1 -> Saturation1/1
  Difference1/1 -> Abs1/1

== system AUAV_V3_TestSensors/Position_and_Attitude_Filter/GPS Update/Detect Change2 ==
  Data : Inport
  Abs1 : Abs  SampleTime=T
  Difference1 : simulink/Discrete/Difference  ICPrevInput=0.0  InputProcessing=Inherited  OutMin=[]  OutMax=[]  OutDataType=sfix(16)  OutScaling=2^-10  DoSatur=off
  Saturation1 : Saturate  UpperLimit=1  LowerLimit=0  SampleTime=T
  change? : Outport
  wires:
  Difference1/1 -> Abs1/1
  Abs1/1 -> Saturation1/1
  Data/1 -> Difference1/1
  Saturation1/1 -> change?/1

== system AUAV_V3_TestSensors/Position_and_Attitude_Filter/Geod2LTP1/ECEF2LTP (UEN) ==
  ECEF coordinates : Inport
  "Long, Lat" : Inport  Port=2
  Deg2R : Gain  Gain=pi/180  SaturateOnIntegerOverflow=on  OutDataTypeStr=Inherit: Same as input  ParamDataTypeStr=Inherit: Same as input
  Demux3 : Demux  Outputs=2
  From Body to Universal1 : Subsystem
  Product1 : Product  Multiplication=Matrix(*)  SaturateOnIntegerOverflow=on  InputSameDT=on  OutDataTypeStr=Inherit: Same as first input
  Out : Outport
  wires:
  From Body to Universal1/1(DCM) -> Product1/1
  ECEF coordinates/1 -> Product1/2
  Deg2R/1 -> Demux3/1
  Demux3/1 -> From Body to Universal1/1(long)
  Demux3/2 -> From Body to Universal1/2(lat)
  Product1/1 -> Out/1
  "Long, Lat"/1 -> Deg2R/1
